simulink model "CryoDetHcd"  (R2016b)
settings: Solver=ode45  StartTime=0.0  StopTime=1e-3  RelTol=1e-3
PreLoadFcn:
  | setup_hcd
values from neighbouring files (symbols this model uses):
  A = sqrt(0.5*erfc(x))    [setup_hcd.m]
  etaRomData = zeros(1,128)    [setup_hcd.m]
  Fadc = 614e6    (= 614000000)    [setup_hcd.m]
  freqRomData = zeros(1,128)    [setup_hcd.m]
  freqRomData1 = zeros(1,128)    [setup_hcd.m]
  freqRomData2 = zeros(1,128)    [setup_hcd.m]
  freqRomData3 = zeros(1,128)    [setup_hcd.m]
undefined symbols (not defined in the file or in its folder): AXI4, B, C, D, j, Lite
libraries: xbsIndex_r4 x2151, CryoDetLibCMB x28, hdlsllib x8, dspsigops x2, simulink x1
(part 16 of 17)

== system CryoDetHcd/DspCore/DSP/channel_processor/channel_processor_x4/128_channel_processor3/Variant Subsystem/LMS/controller/1st_harmonic1/Subsystem1 ==
  note: D=2
  gain : Inport
  in : Inport  Port=2
  Mux : xbsIndex_r4/Mux  inputs=8  en=off  latency=1  precision=Full  arith_type=Unsigned  n_bits=16  bin_pt=14  quantization=Truncate  overflow=Wrap  dbl_ovrd=off  block_type=mux
  Shift2 : xbsIndex_r4/Shift  shift_dir=Right  shift_bits=13  en=off  latency=1  precision=User Defined  arith_type="Signed  (2's comp)"  n_bits=32  bin_pt=32  quantization=Truncate  overflow=Wrap  dbl_ovrd=off  block_type=shift
  Shift3 : xbsIndex_r4/Shift  shift_dir=Right  shift_bits=12  en=off  latency=1  precision=User Defined  arith_type="Signed  (2's comp)"  n_bits=32  bin_pt=32  quantization=Truncate  overflow=Wrap  dbl_ovrd=off  block_type=shift
  Shift4 : xbsIndex_r4/Shift  shift_dir=Right  shift_bits=6  en=off  latency=1  precision=User Defined  arith_type="Signed  (2's comp)"  n_bits=32  bin_pt=32  quantization=Truncate  overflow=Wrap  dbl_ovrd=off  block_type=shift
  Shift5 : xbsIndex_r4/Shift  shift_dir=Right  shift_bits=7  en=off  latency=1  precision=User Defined  arith_type="Signed  (2's comp)"  n_bits=32  bin_pt=32  quantization=Truncate  overflow=Wrap  dbl_ovrd=off  block_type=shift
  Shift6 : xbsIndex_r4/Shift  shift_dir=Right  shift_bits=8  en=off  latency=1  precision=User Defined  arith_type="Signed  (2's comp)"  n_bits=32  bin_pt=32  quantization=Truncate  overflow=Wrap  dbl_ovrd=off  block_type=shift
  Shift7 : xbsIndex_r4/Shift  shift_dir=Right  shift_bits=9  en=off  latency=1  precision=User Defined  arith_type="Signed  (2's comp)"  n_bits=32  bin_pt=32  quantization=Truncate  overflow=Wrap  dbl_ovrd=off  block_type=shift
  Shift8 : xbsIndex_r4/Shift  shift_dir=Right  shift_bits=10  en=off  latency=1  precision=User Defined  arith_type="Signed  (2's comp)"  n_bits=32  bin_pt=32  quantization=Truncate  overflow=Wrap  dbl_ovrd=off  block_type=shift
  Shift9 : xbsIndex_r4/Shift  shift_dir=Right  shift_bits=11  en=off  latency=1  precision=User Defined  arith_type="Signed  (2's comp)"  n_bits=32  bin_pt=32  quantization=Truncate  overflow=Wrap  dbl_ovrd=off  block_type=shift
  out : Outport
  wires:
  Shift4/1 -> Mux/9
  Shift5/1 -> Mux/8
  Shift6/1 -> Mux/7
  Shift7/1 -> Mux/6
  Shift8/1 -> Mux/5
  Shift9/1 -> Mux/4
  Shift3/1 -> Mux/3
  Shift2/1 -> Mux/2
  in/1 -> Shift2/1, Shift3/1, Shift9/1, Shift8/1, Shift7/1, Shift6/1, Shift5/1, Shift4/1
  Mux/1 -> out/1
  gain/1 -> Mux/1

== system CryoDetHcd/DspCore/DSP/channel_processor/channel_processor_x4/128_channel_processor3/Variant Subsystem/LMS/controller/1st_harmonic1/interleaved_accumulator1 ==
  note: D=5
  In1 : Inport
  enable : Inport  Port=2
  AddSub : xbsIndex_r4/AddSub  mode=Addition  use_carryin=off  use_carryout=off  en=off  latency=3  precision=User Defined  arith_type="Signed  (2's comp)"  n_bits=32  bin_pt=32  quantization=Truncate  overflow=Wrap  use_behavioral_HDL=off  hw_selection=Fabric  pipelined=off  dbl_ovrd=off  block_type=addsub
  Constant : xbsIndex_r4/Constant  const=0  gui_display_data_type=Fixed-point  arith_type=Signed (2's comp)  n_bits=32  bin_pt=32  preci_type=Single  exp_width=8  frac_width=24  explicit_period=off  period=1  equ=P=C  opselect=C  inp2=PCIN>>17  opr=+  inp1=P  carry=CIN  dbl_ovrd=off  block_type=constant
  Convert : xbsIndex_r4/Convert  gui_display_data_type=Fixed-point  arith_type="Signed  (2's comp)"  n_bits=28  bin_pt=28  float_type=Single  exp_bits=8  fraction_bits=24  quantization=Truncate  overflow=Wrap  en=off  latency=1  pipeline=off  dbl_ovrd=off  block_type=convert
  Delay : xbsIndex_r4/Delay  rst=off  infoeditControl=Selection of Reset will increase slice count due to use of real FFs and instead of SRLs  en=off  latency=124  reg_retiming=off  dbl_ovrd=off  block_type=delay
  Delay1 : xbsIndex_r4/Delay  rst=off  infoeditControl=Selection of Reset will increase slice count due to use of real FFs and instead of SRLs  en=off  latency=3  reg_retiming=off  dbl_ovrd=off  block_type=delay
  Mux : xbsIndex_r4/Mux  inputs=2  en=off  latency=1  precision=Full  arith_type=Unsigned  n_bits=16  bin_pt=14  quantization=Truncate  overflow=Wrap  dbl_ovrd=off  block_type=mux
  Out1 : Outport
  wires:
  In1/1 -> AddSub/1
  Delay/1 -> AddSub/2
  Convert/1 -> Out1/1
  Mux/1 -> Delay/1, Convert/1
  enable/1 -> Delay1/1
  Constant/1 -> Mux/2
  AddSub/1 -> Mux/3
  Delay1/1 -> Mux/1

== system CryoDetHcd/DspCore/DSP/channel_processor/channel_processor_x4/128_channel_processor3/Variant Subsystem/LMS/controller/1st_harmonic1/interleaved_accumulator2 ==
  In1 : Inport
  enable : Inport  Port=2
  AddSub : xbsIndex_r4/AddSub  mode=Addition  use_carryin=off  use_carryout=off  en=off  latency=3  precision=User Defined  arith_type="Signed  (2's comp)"  n_bits=32  bin_pt=32  quantization=Truncate  overflow=Wrap  use_behavioral_HDL=off  hw_selection=Fabric  pipelined=off  dbl_ovrd=off  block_type=addsub
  Constant : xbsIndex_r4/Constant  const=0  gui_display_data_type=Fixed-point  arith_type=Signed (2's comp)  n_bits=32  bin_pt=32  preci_type=Single  exp_width=8  frac_width=24  explicit_period=off  period=1  equ=P=C  opselect=C  inp2=PCIN>>17  opr=+  inp1=P  carry=CIN  dbl_ovrd=off  block_type=constant
  Convert : xbsIndex_r4/Convert  gui_display_data_type=Fixed-point  arith_type="Signed  (2's comp)"  n_bits=28  bin_pt=28  float_type=Single  exp_bits=8  fraction_bits=24  quantization=Truncate  overflow=Wrap  en=off  latency=1  pipeline=off  dbl_ovrd=off  block_type=convert
  Delay : xbsIndex_r4/Delay  rst=off  infoeditControl=Selection of Reset will increase slice count due to use of real FFs and instead of SRLs  en=off  latency=124  reg_retiming=off  dbl_ovrd=off  block_type=delay
  Delay1 : xbsIndex_r4/Delay  rst=off  infoeditControl=Selection of Reset will increase slice count due to use of real FFs and instead of SRLs  en=off  latency=3  reg_retiming=off  dbl_ovrd=off  block_type=delay
  Mux : xbsIndex_r4/Mux  inputs=2  en=off  latency=1  precision=Full  arith_type=Unsigned  n_bits=16  bin_pt=14  quantization=Truncate  overflow=Wrap  dbl_ovrd=off  block_type=mux
  Out1 : Outport
  wires:
  Delay1/1 -> Mux/1
  AddSub/1 -> Mux/3
  Constant/1 -> Mux/2
  enable/1 -> Delay1/1
  Mux/1 -> Convert/1, Delay/1
  Convert/1 -> Out1/1
  Delay/1 -> AddSub/2
  In1/1 -> AddSub/1

== system CryoDetHcd/DspCore/DSP/channel_processor/channel_processor_x4/128_channel_processor3/Variant Subsystem/LMS/controller/1st_harmonic2/Subsystem ==
  note: D=2
  gain : Inport
  in : Inport  Port=2
  Mux : xbsIndex_r4/Mux  inputs=8  en=off  latency=1  precision=Full  arith_type=Unsigned  n_bits=16  bin_pt=14  quantization=Truncate  overflow=Wrap  dbl_ovrd=off  block_type=mux
  Shift2 : xbsIndex_r4/Shift  shift_dir=Right  shift_bits=13  en=off  latency=1  precision=User Defined  arith_type="Signed  (2's comp)"  n_bits=32  bin_pt=32  quantization=Truncate  overflow=Wrap  dbl_ovrd=off  block_type=shift
  Shift3 : xbsIndex_r4/Shift  shift_dir=Right  shift_bits=12  en=off  latency=1  precision=User Defined  arith_type="Signed  (2's comp)"  n_bits=32  bin_pt=32  quantization=Truncate  overflow=Wrap  dbl_ovrd=off  block_type=shift
  Shift4 : xbsIndex_r4/Shift  shift_dir=Right  shift_bits=6  en=off  latency=1  precision=User Defined  arith_type="Signed  (2's comp)"  n_bits=32  bin_pt=32  quantization=Truncate  overflow=Wrap  dbl_ovrd=off  block_type=shift
  Shift5 : xbsIndex_r4/Shift  shift_dir=Right  shift_bits=7  en=off  latency=1  precision=User Defined  arith_type="Signed  (2's comp)"  n_bits=32  bin_pt=32  quantization=Truncate  overflow=Wrap  dbl_ovrd=off  block_type=shift
  Shift6 : xbsIndex_r4/Shift  shift_dir=Right  shift_bits=8  en=off  latency=1  precision=User Defined  arith_type="Signed  (2's comp)"  n_bits=32  bin_pt=32  quantization=Truncate  overflow=Wrap  dbl_ovrd=off  block_type=shift
  Shift7 : xbsIndex_r4/Shift  shift_dir=Right  shift_bits=9  en=off  latency=1  precision=User Defined  arith_type="Signed  (2's comp)"  n_bits=32  bin_pt=32  quantization=Truncate  overflow=Wrap  dbl_ovrd=off  block_type=shift
  Shift8 : xbsIndex_r4/Shift  shift_dir=Right  shift_bits=10  en=off  latency=1  precision=User Defined  arith_type="Signed  (2's comp)"  n_bits=32  bin_pt=32  quantization=Truncate  overflow=Wrap  dbl_ovrd=off  block_type=shift
  Shift9 : xbsIndex_r4/Shift  shift_dir=Right  shift_bits=11  en=off  latency=1  precision=User Defined  arith_type="Signed  (2's comp)"  n_bits=32  bin_pt=32  quantization=Truncate  overflow=Wrap  dbl_ovrd=off  block_type=shift
  out : Outport
  wires:
  Shift4/1 -> Mux/9
  Shift5/1 -> Mux/8
  Shift6/1 -> Mux/7
  Shift7/1 -> Mux/6
  Shift8/1 -> Mux/5
  Shift9/1 -> Mux/4
  Shift3/1 -> Mux/3
  Shift2/1 -> Mux/2
  in/1 -> Shift2/1, Shift3/1, Shift9/1, Shift8/1, Shift7/1, Shift6/1, Shift5/1, Shift4/1
  Mux/1 -> out/1
  gain/1 -> Mux/1

== system CryoDetHcd/DspCore/DSP/channel_processor/channel_processor_x4/128_channel_processor3/Variant Subsystem/LMS/controller/1st_harmonic2/Subsystem1 ==
  note: D=2
  gain : Inport
  in : Inport  Port=2
  Mux : xbsIndex_r4/Mux  inputs=8  en=off  latency=1  precision=Full  arith_type=Unsigned  n_bits=16  bin_pt=14  quantization=Truncate  overflow=Wrap  dbl_ovrd=off  block_type=mux
  Shift2 : xbsIndex_r4/Shift  shift_dir=Right  shift_bits=13  en=off  latency=1  precision=User Defined  arith_type="Signed  (2's comp)"  n_bits=32  bin_pt=32  quantization=Truncate  overflow=Wrap  dbl_ovrd=off  block_type=shift
  Shift3 : xbsIndex_r4/Shift  shift_dir=Right  shift_bits=12  en=off  latency=1  precision=User Defined  arith_type="Signed  (2's comp)"  n_bits=32  bin_pt=32  quantization=Truncate  overflow=Wrap  dbl_ovrd=off  block_type=shift
  Shift4 : xbsIndex_r4/Shift  shift_dir=Right  shift_bits=6  en=off  latency=1  precision=User Defined  arith_type="Signed  (2's comp)"  n_bits=32  bin_pt=32  quantization=Truncate  overflow=Wrap  dbl_ovrd=off  block_type=shift
  Shift5 : xbsIndex_r4/Shift  shift_dir=Right  shift_bits=7  en=off  latency=1  precision=User Defined  arith_type="Signed  (2's comp)"  n_bits=32  bin_pt=32  quantization=Truncate  overflow=Wrap  dbl_ovrd=off  block_type=shift
  Shift6 : xbsIndex_r4/Shift  shift_dir=Right  shift_bits=8  en=off  latency=1  precision=User Defined  arith_type="Signed  (2's comp)"  n_bits=32  bin_pt=32  quantization=Truncate  overflow=Wrap  dbl_ovrd=off  block_type=shift
  Shift7 : xbsIndex_r4/Shift  shift_dir=Right  shift_bits=9  en=off  latency=1  precision=User Defined  arith_type="Signed  (2's comp)"  n_bits=32  bin_pt=32  quantization=Truncate  overflow=Wrap  dbl_ovrd=off  block_type=shift
  Shift8 : xbsIndex_r4/Shift  shift_dir=Right  shift_bits=10  en=off  latency=1  precision=User Defined  arith_type="Signed  (2's comp)"  n_bits=32  bin_pt=32  quantization=Truncate  overflow=Wrap  dbl_ovrd=off  block_type=shift
  Shift9 : xbsIndex_r4/Shift  shift_dir=Right  shift_bits=11  en=off  latency=1  precision=User Defined  arith_type="Signed  (2's comp)"  n_bits=32  bin_pt=32  quantization=Truncate  overflow=Wrap  dbl_ovrd=off  block_type=shift
  out : Outport
  wires:
  gain/1 -> Mux/1
  Mux/1 -> out/1
  in/1 -> Shift4/1, Shift5/1, Shift6/1, Shift7/1, Shift8/1, Shift9/1, Shift3/1, Shift2/1
  Shift2/1 -> Mux/2
  Shift3/1 -> Mux/3
  Shift9/1 -> Mux/4
  Shift8/1 -> Mux/5
  Shift7/1 -> Mux/6
  Shift6/1 -> Mux/7
  Shift5/1 -> Mux/8
  Shift4/1 -> Mux/9

== system CryoDetHcd/DspCore/DSP/channel_processor/channel_processor_x4/128_channel_processor3/Variant Subsystem/LMS/controller/1st_harmonic2/interleaved_accumulator1 ==
  note: D=5
  In1 : Inport
  enable : Inport  Port=2
  AddSub : xbsIndex_r4/AddSub  mode=Addition  use_carryin=off  use_carryout=off  en=off  latency=3  precision=User Defined  arith_type="Signed  (2's comp)"  n_bits=32  bin_pt=32  quantization=Truncate  overflow=Wrap  use_behavioral_HDL=off  hw_selection=Fabric  pipelined=off  dbl_ovrd=off  block_type=addsub
  Constant : xbsIndex_r4/Constant  const=0  gui_display_data_type=Fixed-point  arith_type=Signed (2's comp)  n_bits=32  bin_pt=32  preci_type=Single  exp_width=8  frac_width=24  explicit_period=off  period=1  equ=P=C  opselect=C  inp2=PCIN>>17  opr=+  inp1=P  carry=CIN  dbl_ovrd=off  block_type=constant
  Convert : xbsIndex_r4/Convert  gui_display_data_type=Fixed-point  arith_type="Signed  (2's comp)"  n_bits=28  bin_pt=28  float_type=Single  exp_bits=8  fraction_bits=24  quantization=Truncate  overflow=Wrap  en=off  latency=1  pipeline=off  dbl_ovrd=off  block_type=convert
  Delay : xbsIndex_r4/Delay  rst=off  infoeditControl=Selection of Reset will increase slice count due to use of real FFs and instead of SRLs  en=off  latency=124  reg_retiming=off  dbl_ovrd=off  block_type=delay
  Delay1 : xbsIndex_r4/Delay  rst=off  infoeditControl=Selection of Reset will increase slice count due to use of real FFs and instead of SRLs  en=off  latency=3  reg_retiming=off  dbl_ovrd=off  block_type=delay
  Mux : xbsIndex_r4/Mux  inputs=2  en=off  latency=1  precision=Full  arith_type=Unsigned  n_bits=16  bin_pt=14  quantization=Truncate  overflow=Wrap  dbl_ovrd=off  block_type=mux
  Out1 : Outport
  wires:
  Delay1/1 -> Mux/1
  AddSub/1 -> Mux/3
  Constant/1 -> Mux/2
  enable/1 -> Delay1/1
  Mux/1 -> Convert/1, Delay/1
  Convert/1 -> Out1/1
  Delay/1 -> AddSub/2
  In1/1 -> AddSub/1

== system CryoDetHcd/DspCore/DSP/channel_processor/channel_processor_x4/128_channel_processor3/Variant Subsystem/LMS/controller/1st_harmonic2/interleaved_accumulator2 ==
  In1 : Inport
  enable : Inport  Port=2
  AddSub : xbsIndex_r4/AddSub  mode=Addition  use_carryin=off  use_carryout=off  en=off  latency=3  precision=User Defined  arith_type="Signed  (2's comp)"  n_bits=32  bin_pt=32  quantization=Truncate  overflow=Wrap  use_behavioral_HDL=off  hw_selection=Fabric  pipelined=off  dbl_ovrd=off  block_type=addsub
  Constant : xbsIndex_r4/Constant  const=0  gui_display_data_type=Fixed-point  arith_type=Signed (2's comp)  n_bits=32  bin_pt=32  preci_type=Single  exp_width=8  frac_width=24  explicit_period=off  period=1  equ=P=C  opselect=C  inp2=PCIN>>17  opr=+  inp1=P  carry=CIN  dbl_ovrd=off  block_type=constant
  Convert : xbsIndex_r4/Convert  gui_display_data_type=Fixed-point  arith_type="Signed  (2's comp)"  n_bits=28  bin_pt=28  float_type=Single  exp_bits=8  fraction_bits=24  quantization=Truncate  overflow=Wrap  en=off  latency=1  pipeline=off  dbl_ovrd=off  block_type=convert
  Delay : xbsIndex_r4/Delay  rst=off  infoeditControl=Selection of Reset will increase slice count due to use of real FFs and instead of SRLs  en=off  latency=124  reg_retiming=off  dbl_ovrd=off  block_type=delay
  Delay1 : xbsIndex_r4/Delay  rst=off  infoeditControl=Selection of Reset will increase slice count due to use of real FFs and instead of SRLs  en=off  latency=3  reg_retiming=off  dbl_ovrd=off  block_type=delay
  Mux : xbsIndex_r4/Mux  inputs=2  en=off  latency=1  precision=Full  arith_type=Unsigned  n_bits=16  bin_pt=14  quantization=Truncate  overflow=Wrap  dbl_ovrd=off  block_type=mux
  Out1 : Outport
  wires:
  In1/1 -> AddSub/1
  Delay/1 -> AddSub/2
  Convert/1 -> Out1/1
  Mux/1 -> Delay/1, Convert/1
  enable/1 -> Delay1/1
  Constant/1 -> Mux/2
  AddSub/1 -> Mux/3
  Delay1/1 -> Mux/1

== system CryoDetHcd/DspCore/DSP/channel_processor/channel_processor_x4/128_channel_processor3/Variant Subsystem/LMS/controller/DC/Subsystem ==
  note: D=2
  gain : Inport
  in : Inport  Port=2
  Mux : xbsIndex_r4/Mux  inputs=8  en=off  latency=1  precision=Full  arith_type=Unsigned  n_bits=16  bin_pt=14  quantization=Truncate  overflow=Wrap  dbl_ovrd=off  block_type=mux
  Shift2 : xbsIndex_r4/Shift  shift_dir=Right  shift_bits=13  en=off  latency=1  precision=User Defined  arith_type="Signed  (2's comp)"  n_bits=32  bin_pt=32  quantization=Truncate  overflow=Wrap  dbl_ovrd=off  block_type=shift
  Shift3 : xbsIndex_r4/Shift  shift_dir=Right  shift_bits=12  en=off  latency=1  precision=User Defined  arith_type="Signed  (2's comp)"  n_bits=32  bin_pt=32  quantization=Truncate  overflow=Wrap  dbl_ovrd=off  block_type=shift
  Shift4 : xbsIndex_r4/Shift  shift_dir=Right  shift_bits=6  en=off  latency=1  precision=User Defined  arith_type="Signed  (2's comp)"  n_bits=32  bin_pt=32  quantization=Truncate  overflow=Wrap  dbl_ovrd=off  block_type=shift
  Shift5 : xbsIndex_r4/Shift  shift_dir=Right  shift_bits=7  en=off  latency=1  precision=User Defined  arith_type="Signed  (2's comp)"  n_bits=32  bin_pt=32  quantization=Truncate  overflow=Wrap  dbl_ovrd=off  block_type=shift
  Shift6 : xbsIndex_r4/Shift  shift_dir=Right  shift_bits=8  en=off  latency=1  precision=User Defined  arith_type="Signed  (2's comp)"  n_bits=32  bin_pt=32  quantization=Truncate  overflow=Wrap  dbl_ovrd=off  block_type=shift
  Shift7 : xbsIndex_r4/Shift  shift_dir=Right  shift_bits=9  en=off  latency=1  precision=User Defined  arith_type="Signed  (2's comp)"  n_bits=32  bin_pt=32  quantization=Truncate  overflow=Wrap  dbl_ovrd=off  block_type=shift
  Shift8 : xbsIndex_r4/Shift  shift_dir=Right  shift_bits=10  en=off  latency=1  precision=User Defined  arith_type="Signed  (2's comp)"  n_bits=32  bin_pt=32  quantization=Truncate  overflow=Wrap  dbl_ovrd=off  block_type=shift
  Shift9 : xbsIndex_r4/Shift  shift_dir=Right  shift_bits=11  en=off  latency=1  precision=User Defined  arith_type="Signed  (2's comp)"  n_bits=32  bin_pt=32  quantization=Truncate  overflow=Wrap  dbl_ovrd=off  block_type=shift
  out : Outport
  wires:
  Shift4/1 -> Mux/9
  Shift5/1 -> Mux/8
  Shift6/1 -> Mux/7
  Shift7/1 -> Mux/6
  Shift8/1 -> Mux/5
  Shift9/1 -> Mux/4
  Shift3/1 -> Mux/3
  Shift2/1 -> Mux/2
  in/1 -> Shift2/1, Shift3/1, Shift9/1, Shift8/1, Shift7/1, Shift6/1, Shift5/1, Shift4/1
  Mux/1 -> out/1
  gain/1 -> Mux/1

== system CryoDetHcd/DspCore/DSP/channel_processor/channel_processor_x4/128_channel_processor3/Variant Subsystem/LMS/controller/DC/interleaved_accumulator2 ==
  In1 : Inport
  enable : Inport  Port=2
  AddSub : xbsIndex_r4/AddSub  mode=Addition  use_carryin=off  use_carryout=off  en=off  latency=3  precision=User Defined  arith_type="Signed  (2's comp)"  n_bits=32  bin_pt=32  quantization=Truncate  overflow=Wrap  use_behavioral_HDL=off  hw_selection=Fabric  pipelined=off  dbl_ovrd=off  block_type=addsub
  Constant : xbsIndex_r4/Constant  const=0  gui_display_data_type=Fixed-point  arith_type=Signed (2's comp)  n_bits=32  bin_pt=32  preci_type=Single  exp_width=8  frac_width=24  explicit_period=off  period=1  equ=P=C  opselect=C  inp2=PCIN>>17  opr=+  inp1=P  carry=CIN  dbl_ovrd=off  block_type=constant
  Convert : xbsIndex_r4/Convert  gui_display_data_type=Fixed-point  arith_type="Signed  (2's comp)"  n_bits=28  bin_pt=28  float_type=Single  exp_bits=8  fraction_bits=24  quantization=Truncate  overflow=Wrap  en=off  latency=1  pipeline=off  dbl_ovrd=off  block_type=convert
  Delay : xbsIndex_r4/Delay  rst=off  infoeditControl=Selection of Reset will increase slice count due to use of real FFs and instead of SRLs  en=off  latency=124  reg_retiming=off  dbl_ovrd=off  block_type=delay
  Delay1 : xbsIndex_r4/Delay  rst=off  infoeditControl=Selection of Reset will increase slice count due to use of real FFs and instead of SRLs  en=off  latency=3  reg_retiming=off  dbl_ovrd=off  block_type=delay
  Mux : xbsIndex_r4/Mux  inputs=2  en=off  latency=1  precision=Full  arith_type=Unsigned  n_bits=16  bin_pt=14  quantization=Truncate  overflow=Wrap  dbl_ovrd=off  block_type=mux
  Out1 : Outport
  wires:
  In1/1 -> AddSub/1
  Delay/1 -> AddSub/2
  Convert/1 -> Out1/1
  Mux/1 -> Delay/1, Convert/1
  enable/1 -> Delay1/1
  Constant/1 -> Mux/2
  AddSub/1 -> Mux/3
  Delay1/1 -> Mux/1

== system CryoDetHcd/DspCore/DSP/channel_processor/channel_processor_x4/128_channel_processor3/Variant Subsystem/LMS/controller/freqs/Subsystem ==
  Chan : Inport
  In2 : Inport  Port=2
  In3 : Inport  Port=3
  In4 : Inport  Port=4
  valid : Inport  Port=5
  Logical : xbsIndex_r4/Logical  logical_function=AND  inputs=2  en=off  latency=0  precision=Full  arith_type=Unsigned  n_bits=16  bin_pt=0  align_bp=on  dbl_ovrd=off  block_type=logical
  Register17 : xbsIndex_r4/Register  init=0  rst=off  en=on  dbl_ovrd=off  block_type=register
  Register18 : xbsIndex_r4/Register  init=0  rst=off  en=on  dbl_ovrd=off  block_type=register
  Relational : xbsIndex_r4/Relational  mode=a=b  op_type=Bool  en=off  latency=0  dbl_ovrd=off  block_type=relational
  Out2 : Outport
  Out3 : Outport  Port=2
  wires:
  Logical/1 -> Register17/2, Register18/2
  valid/1 -> Logical/2
  Relational/1 -> Logical/1
  In3/1 -> Register17/1
  In2/1 -> Relational/2
  Chan/1 -> Relational/1
  Register17/1 -> Out2/1
  Register18/1 -> Out3/1
  In4/1 -> Register18/1

== system CryoDetHcd/DspCore/DSP/channel_processor/channel_processor_x4/128_channel_processor3/Variant Subsystem/LMS/controller/freqs/Subsystem1 ==
  Chan : Inport
  In2 : Inport  Port=2
  In3 : Inport  Port=3
  In4 : Inport  Port=4
  valid : Inport  Port=5
  Logical : xbsIndex_r4/Logical  logical_function=AND  inputs=2  en=off  latency=0  precision=Full  arith_type=Unsigned  n_bits=16  bin_pt=0  align_bp=on  dbl_ovrd=off  block_type=logical
  Register17 : xbsIndex_r4/Register  init=0  rst=off  en=on  dbl_ovrd=off  block_type=register
  Register18 : xbsIndex_r4/Register  init=0  rst=off  en=on  dbl_ovrd=off  block_type=register
  Relational : xbsIndex_r4/Relational  mode=a=b  op_type=Bool  en=off  latency=0  dbl_ovrd=off  block_type=relational
  Out2 : Outport
  Out3 : Outport  Port=2
  wires:
  In4/1 -> Register18/1
  Register18/1 -> Out3/1
  Register17/1 -> Out2/1
  Chan/1 -> Relational/1
  In2/1 -> Relational/2
  In3/1 -> Register17/1
  Relational/1 -> Logical/1
  valid/1 -> Logical/2
  Logical/1 -> Register18/2, Register17/2

== system CryoDetHcd/DspCore/DSP/channel_processor/channel_processor_x4/128_channel_processor3/Variant Subsystem/LMS/controller/freqs/Subsystem2 ==
  Chan : Inport
  In2 : Inport  Port=2
  In3 : Inport  Port=3
  In4 : Inport  Port=4
  valid : Inport  Port=5
  Logical : xbsIndex_r4/Logical  logical_function=AND  inputs=2  en=off  latency=0  precision=Full  arith_type=Unsigned  n_bits=16  bin_pt=0  align_bp=on  dbl_ovrd=off  block_type=logical
  Register17 : xbsIndex_r4/Register  init=0  rst=off  en=on  dbl_ovrd=off  block_type=register
  Register18 : xbsIndex_r4/Register  init=0  rst=off  en=on  dbl_ovrd=off  block_type=register
  Relational : xbsIndex_r4/Relational  mode=a=b  op_type=Bool  en=off  latency=0  dbl_ovrd=off  block_type=relational
  Out2 : Outport
  Out3 : Outport  Port=2
  wires:
  Logical/1 -> Register17/2, Register18/2
  valid/1 -> Logical/2
  Relational/1 -> Logical/1
  In3/1 -> Register17/1
  In2/1 -> Relational/2
  Chan/1 -> Relational/1
  Register17/1 -> Out2/1
  Register18/1 -> Out3/1
  In4/1 -> Register18/1

== system CryoDetHcd/DspCore/DSP/channel_processor/channel_processor_x4/128_channel_processor4/Variant Subsystem/LMS/controller/1st_harmonic/Subsystem ==
  note: D=2
  gain : Inport
  in : Inport  Port=2
  Mux : xbsIndex_r4/Mux  inputs=8  en=off  latency=1  precision=Full  arith_type=Unsigned  n_bits=16  bin_pt=14  quantization=Truncate  overflow=Wrap  dbl_ovrd=off  block_type=mux
  Shift2 : xbsIndex_r4/Shift  shift_dir=Right  shift_bits=13  en=off  latency=1  precision=User Defined  arith_type="Signed  (2's comp)"  n_bits=32  bin_pt=32  quantization=Truncate  overflow=Wrap  dbl_ovrd=off  block_type=shift
  Shift3 : xbsIndex_r4/Shift  shift_dir=Right  shift_bits=12  en=off  latency=1  precision=User Defined  arith_type="Signed  (2's comp)"  n_bits=32  bin_pt=32  quantization=Truncate  overflow=Wrap  dbl_ovrd=off  block_type=shift
  Shift4 : xbsIndex_r4/Shift  shift_dir=Right  shift_bits=6  en=off  latency=1  precision=User Defined  arith_type="Signed  (2's comp)"  n_bits=32  bin_pt=32  quantization=Truncate  overflow=Wrap  dbl_ovrd=off  block_type=shift
  Shift5 : xbsIndex_r4/Shift  shift_dir=Right  shift_bits=7  en=off  latency=1  precision=User Defined  arith_type="Signed  (2's comp)"  n_bits=32  bin_pt=32  quantization=Truncate  overflow=Wrap  dbl_ovrd=off  block_type=shift
  Shift6 : xbsIndex_r4/Shift  shift_dir=Right  shift_bits=8  en=off  latency=1  precision=User Defined  arith_type="Signed  (2's comp)"  n_bits=32  bin_pt=32  quantization=Truncate  overflow=Wrap  dbl_ovrd=off  block_type=shift
  Shift7 : xbsIndex_r4/Shift  shift_dir=Right  shift_bits=9  en=off  latency=1  precision=User Defined  arith_type="Signed  (2's comp)"  n_bits=32  bin_pt=32  quantization=Truncate  overflow=Wrap  dbl_ovrd=off  block_type=shift
  Shift8 : xbsIndex_r4/Shift  shift_dir=Right  shift_bits=10  en=off  latency=1  precision=User Defined  arith_type="Signed  (2's comp)"  n_bits=32  bin_pt=32  quantization=Truncate  overflow=Wrap  dbl_ovrd=off  block_type=shift
  Shift9 : xbsIndex_r4/Shift  shift_dir=Right  shift_bits=11  en=off  latency=1  precision=User Defined  arith_type="Signed  (2's comp)"  n_bits=32  bin_pt=32  quantization=Truncate  overflow=Wrap  dbl_ovrd=off  block_type=shift
  out : Outport
  wires:
  gain/1 -> Mux/1
  Mux/1 -> out/1
  in/1 -> Shift4/1, Shift5/1, Shift6/1, Shift7/1, Shift8/1, Shift9/1, Shift3/1, Shift2/1
  Shift2/1 -> Mux/2
  Shift3/1 -> Mux/3
  Shift9/1 -> Mux/4
  Shift8/1 -> Mux/5
  Shift7/1 -> Mux/6
  Shift6/1 -> Mux/7
  Shift5/1 -> Mux/8
  Shift4/1 -> Mux/9

== system CryoDetHcd/DspCore/DSP/channel_processor/channel_processor_x4/128_channel_processor4/Variant Subsystem/LMS/controller/1st_harmonic/Subsystem1 ==
  note: D=2
  gain : Inport
  in : Inport  Port=2
  Mux : xbsIndex_r4/Mux  inputs=8  en=off  latency=1  precision=Full  arith_type=Unsigned  n_bits=16  bin_pt=14  quantization=Truncate  overflow=Wrap  dbl_ovrd=off  block_type=mux
  Shift2 : xbsIndex_r4/Shift  shift_dir=Right  shift_bits=13  en=off  latency=1  precision=User Defined  arith_type="Signed  (2's comp)"  n_bits=32  bin_pt=32  quantization=Truncate  overflow=Wrap  dbl_ovrd=off  block_type=shift
  Shift3 : xbsIndex_r4/Shift  shift_dir=Right  shift_bits=12  en=off  latency=1  precision=User Defined  arith_type="Signed  (2's comp)"  n_bits=32  bin_pt=32  quantization=Truncate  overflow=Wrap  dbl_ovrd=off  block_type=shift
  Shift4 : xbsIndex_r4/Shift  shift_dir=Right  shift_bits=6  en=off  latency=1  precision=User Defined  arith_type="Signed  (2's comp)"  n_bits=32  bin_pt=32  quantization=Truncate  overflow=Wrap  dbl_ovrd=off  block_type=shift
  Shift5 : xbsIndex_r4/Shift  shift_dir=Right  shift_bits=7  en=off  latency=1  precision=User Defined  arith_type="Signed  (2's comp)"  n_bits=32  bin_pt=32  quantization=Truncate  overflow=Wrap  dbl_ovrd=off  block_type=shift
  Shift6 : xbsIndex_r4/Shift  shift_dir=Right  shift_bits=8  en=off  latency=1  precision=User Defined  arith_type="Signed  (2's comp)"  n_bits=32  bin_pt=32  quantization=Truncate  overflow=Wrap  dbl_ovrd=off  block_type=shift
  Shift7 : xbsIndex_r4/Shift  shift_dir=Right  shift_bits=9  en=off  latency=1  precision=User Defined  arith_type="Signed  (2's comp)"  n_bits=32  bin_pt=32  quantization=Truncate  overflow=Wrap  dbl_ovrd=off  block_type=shift
  Shift8 : xbsIndex_r4/Shift  shift_dir=Right  shift_bits=10  en=off  latency=1  precision=User Defined  arith_type="Signed  (2's comp)"  n_bits=32  bin_pt=32  quantization=Truncate  overflow=Wrap  dbl_ovrd=off  block_type=shift
  Shift9 : xbsIndex_r4/Shift  shift_dir=Right  shift_bits=11  en=off  latency=1  precision=User Defined  arith_type="Signed  (2's comp)"  n_bits=32  bin_pt=32  quantization=Truncate  overflow=Wrap  dbl_ovrd=off  block_type=shift
  out : Outport
  wires:
  Shift4/1 -> Mux/9
  Shift5/1 -> Mux/8
  Shift6/1 -> Mux/7
  Shift7/1 -> Mux/6
  Shift8/1 -> Mux/5
  Shift9/1 -> Mux/4
  Shift3/1 -> Mux/3
  Shift2/1 -> Mux/2
  in/1 -> Shift2/1, Shift3/1, Shift9/1, Shift8/1, Shift7/1, Shift6/1, Shift5/1, Shift4/1
  Mux/1 -> out/1
  gain/1 -> Mux/1

== system CryoDetHcd/DspCore/DSP/channel_processor/channel_processor_x4/128_channel_processor4/Variant Subsystem/LMS/controller/1st_harmonic/interleaved_accumulator1 ==
  note: D=5
  In1 : Inport
  enable : Inport  Port=2
  AddSub : xbsIndex_r4/AddSub  mode=Addition  use_carryin=off  use_carryout=off  en=off  latency=3  precision=User Defined  arith_type="Signed  (2's comp)"  n_bits=32  bin_pt=32  quantization=Truncate  overflow=Wrap  use_behavioral_HDL=off  hw_selection=Fabric  pipelined=off  dbl_ovrd=off  block_type=addsub
  Constant : xbsIndex_r4/Constant  const=0  gui_display_data_type=Fixed-point  arith_type=Signed (2's comp)  n_bits=32  bin_pt=32  preci_type=Single  exp_width=8  frac_width=24  explicit_period=off  period=1  equ=P=C  opselect=C  inp2=PCIN>>17  opr=+  inp1=P  carry=CIN  dbl_ovrd=off  block_type=constant
  Convert : xbsIndex_r4/Convert  gui_display_data_type=Fixed-point  arith_type="Signed  (2's comp)"  n_bits=28  bin_pt=28  float_type=Single  exp_bits=8  fraction_bits=24  quantization=Truncate  overflow=Wrap  en=off  latency=1  pipeline=off  dbl_ovrd=off  block_type=convert
  Delay : xbsIndex_r4/Delay  rst=off  infoeditControl=Selection of Reset will increase slice count due to use of real FFs and instead of SRLs  en=off  latency=124  reg_retiming=off  dbl_ovrd=off  block_type=delay
  Delay1 : xbsIndex_r4/Delay  rst=off  infoeditControl=Selection of Reset will increase slice count due to use of real FFs and instead of SRLs  en=off  latency=3  reg_retiming=off  dbl_ovrd=off  block_type=delay
  Mux : xbsIndex_r4/Mux  inputs=2  en=off  latency=1  precision=Full  arith_type=Unsigned  n_bits=16  bin_pt=14  quantization=Truncate  overflow=Wrap  dbl_ovrd=off  block_type=mux
  Out1 : Outport
  wires:
  In1/1 -> AddSub/1
  Delay/1 -> AddSub/2
  Convert/1 -> Out1/1
  Mux/1 -> Delay/1, Convert/1
  enable/1 -> Delay1/1
  Constant/1 -> Mux/2
  AddSub/1 -> Mux/3
  Delay1/1 -> Mux/1

== system CryoDetHcd/DspCore/DSP/channel_processor/channel_processor_x4/128_channel_processor4/Variant Subsystem/LMS/controller/1st_harmonic/interleaved_accumulator2 ==
  In1 : Inport
  enable : Inport  Port=2
  AddSub : xbsIndex_r4/AddSub  mode=Addition  use_carryin=off  use_carryout=off  en=off  latency=3  precision=User Defined  arith_type="Signed  (2's comp)"  n_bits=32  bin_pt=32  quantization=Truncate  overflow=Wrap  use_behavioral_HDL=off  hw_selection=Fabric  pipelined=off  dbl_ovrd=off  block_type=addsub
  Constant : xbsIndex_r4/Constant  const=0  gui_display_data_type=Fixed-point  arith_type=Signed (2's comp)  n_bits=32  bin_pt=32  preci_type=Single  exp_width=8  frac_width=24  explicit_period=off  period=1  equ=P=C  opselect=C  inp2=PCIN>>17  opr=+  inp1=P  carry=CIN  dbl_ovrd=off  block_type=constant
  Convert : xbsIndex_r4/Convert  gui_display_data_type=Fixed-point  arith_type="Signed  (2's comp)"  n_bits=28  bin_pt=28  float_type=Single  exp_bits=8  fraction_bits=24  quantization=Truncate  overflow=Wrap  en=off  latency=1  pipeline=off  dbl_ovrd=off  block_type=convert
  Delay : xbsIndex_r4/Delay  rst=off  infoeditControl=Selection of Reset will increase slice count due to use of real FFs and instead of SRLs  en=off  latency=124  reg_retiming=off  dbl_ovrd=off  block_type=delay
  Delay1 : xbsIndex_r4/Delay  rst=off  infoeditControl=Selection of Reset will increase slice count due to use of real FFs and instead of SRLs  en=off  latency=3  reg_retiming=off  dbl_ovrd=off  block_type=delay
  Mux : xbsIndex_r4/Mux  inputs=2  en=off  latency=1  precision=Full  arith_type=Unsigned  n_bits=16  bin_pt=14  quantization=Truncate  overflow=Wrap  dbl_ovrd=off  block_type=mux
  Out1 : Outport
  wires:
  Delay1/1 -> Mux/1
  AddSub/1 -> Mux/3
  Constant/1 -> Mux/2
  enable/1 -> Delay1/1
  Mux/1 -> Convert/1, Delay/1
  Convert/1 -> Out1/1
  Delay/1 -> AddSub/2
  In1/1 -> AddSub/1

== system CryoDetHcd/DspCore/DSP/channel_processor/channel_processor_x4/128_channel_processor4/Variant Subsystem/LMS/controller/1st_harmonic1/Subsystem ==
  note: D=2
  gain : Inport
  in : Inport  Port=2
  Mux : xbsIndex_r4/Mux  inputs=8  en=off  latency=1  precision=Full  arith_type=Unsigned  n_bits=16  bin_pt=14  quantization=Truncate  overflow=Wrap  dbl_ovrd=off  block_type=mux
  Shift2 : xbsIndex_r4/Shift  shift_dir=Right  shift_bits=13  en=off  latency=1  precision=User Defined  arith_type="Signed  (2's comp)"  n_bits=32  bin_pt=32  quantization=Truncate  overflow=Wrap  dbl_ovrd=off  block_type=shift
  Shift3 : xbsIndex_r4/Shift  shift_dir=Right  shift_bits=12  en=off  latency=1  precision=User Defined  arith_type="Signed  (2's comp)"  n_bits=32  bin_pt=32  quantization=Truncate  overflow=Wrap  dbl_ovrd=off  block_type=shift
  Shift4 : xbsIndex_r4/Shift  shift_dir=Right  shift_bits=6  en=off  latency=1  precision=User Defined  arith_type="Signed  (2's comp)"  n_bits=32  bin_pt=32  quantization=Truncate  overflow=Wrap  dbl_ovrd=off  block_type=shift
  Shift5 : xbsIndex_r4/Shift  shift_dir=Right  shift_bits=7  en=off  latency=1  precision=User Defined  arith_type="Signed  (2's comp)"  n_bits=32  bin_pt=32  quantization=Truncate  overflow=Wrap  dbl_ovrd=off  block_type=shift
  Shift6 : xbsIndex_r4/Shift  shift_dir=Right  shift_bits=8  en=off  latency=1  precision=User Defined  arith_type="Signed  (2's comp)"  n_bits=32  bin_pt=32  quantization=Truncate  overflow=Wrap  dbl_ovrd=off  block_type=shift
  Shift7 : xbsIndex_r4/Shift  shift_dir=Right  shift_bits=9  en=off  latency=1  precision=User Defined  arith_type="Signed  (2's comp)"  n_bits=32  bin_pt=32  quantization=Truncate  overflow=Wrap  dbl_ovrd=off  block_type=shift
  Shift8 : xbsIndex_r4/Shift  shift_dir=Right  shift_bits=10  en=off  latency=1  precision=User Defined  arith_type="Signed  (2's comp)"  n_bits=32  bin_pt=32  quantization=Truncate  overflow=Wrap  dbl_ovrd=off  block_type=shift
  Shift9 : xbsIndex_r4/Shift  shift_dir=Right  shift_bits=11  en=off  latency=1  precision=User Defined  arith_type="Signed  (2's comp)"  n_bits=32  bin_pt=32  quantization=Truncate  overflow=Wrap  dbl_ovrd=off  block_type=shift
  out : Outport
  wires:
  Shift4/1 -> Mux/9
  Shift5/1 -> Mux/8
  Shift6/1 -> Mux/7
  Shift7/1 -> Mux/6
  Shift8/1 -> Mux/5
  Shift9/1 -> Mux/4
  Shift3/1 -> Mux/3
  Shift2/1 -> Mux/2
  in/1 -> Shift2/1, Shift3/1, Shift9/1, Shift8/1, Shift7/1, Shift6/1, Shift5/1, Shift4/1
  Mux/1 -> out/1
  gain/1 -> Mux/1

== system CryoDetHcd/DspCore/DSP/channel_processor/channel_processor_x4/128_channel_processor4/Variant Subsystem/LMS/controller/1st_harmonic1/Subsystem1 ==
  note: D=2
  gain : Inport
  in : Inport  Port=2
  Mux : xbsIndex_r4/Mux  inputs=8  en=off  latency=1  precision=Full  arith_type=Unsigned  n_bits=16  bin_pt=14  quantization=Truncate  overflow=Wrap  dbl_ovrd=off  block_type=mux
  Shift2 : xbsIndex_r4/Shift  shift_dir=Right  shift_bits=13  en=off  latency=1  precision=User Defined  arith_type="Signed  (2's comp)"  n_bits=32  bin_pt=32  quantization=Truncate  overflow=Wrap  dbl_ovrd=off  block_type=shift
  Shift3 : xbsIndex_r4/Shift  shift_dir=Right  shift_bits=12  en=off  latency=1  precision=User Defined  arith_type="Signed  (2's comp)"  n_bits=32  bin_pt=32  quantization=Truncate  overflow=Wrap  dbl_ovrd=off  block_type=shift
  Shift4 : xbsIndex_r4/Shift  shift_dir=Right  shift_bits=6  en=off  latency=1  precision=User Defined  arith_type="Signed  (2's comp)"  n_bits=32  bin_pt=32  quantization=Truncate  overflow=Wrap  dbl_ovrd=off  block_type=shift
  Shift5 : xbsIndex_r4/Shift  shift_dir=Right  shift_bits=7  en=off  latency=1  precision=User Defined  arith_type="Signed  (2's comp)"  n_bits=32  bin_pt=32  quantization=Truncate  overflow=Wrap  dbl_ovrd=off  block_type=shift
  Shift6 : xbsIndex_r4/Shift  shift_dir=Right  shift_bits=8  en=off  latency=1  precision=User Defined  arith_type="Signed  (2's comp)"  n_bits=32  bin_pt=32  quantization=Truncate  overflow=Wrap  dbl_ovrd=off  block_type=shift
  Shift7 : xbsIndex_r4/Shift  shift_dir=Right  shift_bits=9  en=off  latency=1  precision=User Defined  arith_type="Signed  (2's comp)"  n_bits=32  bin_pt=32  quantization=Truncate  overflow=Wrap  dbl_ovrd=off  block_type=shift
  Shift8 : xbsIndex_r4/Shift  shift_dir=Right  shift_bits=10  en=off  latency=1  precision=User Defined  arith_type="Signed  (2's comp)"  n_bits=32  bin_pt=32  quantization=Truncate  overflow=Wrap  dbl_ovrd=off  block_type=shift
  Shift9 : xbsIndex_r4/Shift  shift_dir=Right  shift_bits=11  en=off  latency=1  precision=User Defined  arith_type="Signed  (2's comp)"  n_bits=32  bin_pt=32  quantization=Truncate  overflow=Wrap  dbl_ovrd=off  block_type=shift
  out : Outport
  wires:
  gain/1 -> Mux/1
  Mux/1 -> out/1
  in/1 -> Shift4/1, Shift5/1, Shift6/1, Shift7/1, Shift8/1, Shift9/1, Shift3/1, Shift2/1
  Shift2/1 -> Mux/2
  Shift3/1 -> Mux/3
  Shift9/1 -> Mux/4
  Shift8/1 -> Mux/5
  Shift7/1 -> Mux/6
  Shift6/1 -> Mux/7
  Shift5/1 -> Mux/8
  Shift4/1 -> Mux/9

== system CryoDetHcd/DspCore/DSP/channel_processor/channel_processor_x4/128_channel_processor4/Variant Subsystem/LMS/controller/1st_harmonic1/interleaved_accumulator1 ==
  note: D=5
  In1 : Inport
  enable : Inport  Port=2
  AddSub : xbsIndex_r4/AddSub  mode=Addition  use_carryin=off  use_carryout=off  en=off  latency=3  precision=User Defined  arith_type="Signed  (2's comp)"  n_bits=32  bin_pt=32  quantization=Truncate  overflow=Wrap  use_behavioral_HDL=off  hw_selection=Fabric  pipelined=off  dbl_ovrd=off  block_type=addsub
  Constant : xbsIndex_r4/Constant  const=0  gui_display_data_type=Fixed-point  arith_type=Signed (2's comp)  n_bits=32  bin_pt=32  preci_type=Single  exp_width=8  frac_width=24  explicit_period=off  period=1  equ=P=C  opselect=C  inp2=PCIN>>17  opr=+  inp1=P  carry=CIN  dbl_ovrd=off  block_type=constant
  Convert : xbsIndex_r4/Convert  gui_display_data_type=Fixed-point  arith_type="Signed  (2's comp)"  n_bits=28  bin_pt=28  float_type=Single  exp_bits=8  fraction_bits=24  quantization=Truncate  overflow=Wrap  en=off  latency=1  pipeline=off  dbl_ovrd=off  block_type=convert
  Delay : xbsIndex_r4/Delay  rst=off  infoeditControl=Selection of Reset will increase slice count due to use of real FFs and instead of SRLs  en=off  latency=124  reg_retiming=off  dbl_ovrd=off  block_type=delay
  Delay1 : xbsIndex_r4/Delay  rst=off  infoeditControl=Selection of Reset will increase slice count due to use of real FFs and instead of SRLs  en=off  latency=3  reg_retiming=off  dbl_ovrd=off  block_type=delay
  Mux : xbsIndex_r4/Mux  inputs=2  en=off  latency=1  precision=Full  arith_type=Unsigned  n_bits=16  bin_pt=14  quantization=Truncate  overflow=Wrap  dbl_ovrd=off  block_type=mux
  Out1 : Outport
  wires:
  Delay1/1 -> Mux/1
  AddSub/1 -> Mux/3
  Constant/1 -> Mux/2
  enable/1 -> Delay1/1
  Mux/1 -> Convert/1, Delay/1
  Convert/1 -> Out1/1
  Delay/1 -> AddSub/2
  In1/1 -> AddSub/1

== system CryoDetHcd/DspCore/DSP/channel_processor/channel_processor_x4/128_channel_processor4/Variant Subsystem/LMS/controller/1st_harmonic1/interleaved_accumulator2 ==
  In1 : Inport
  enable : Inport  Port=2
  AddSub : xbsIndex_r4/AddSub  mode=Addition  use_carryin=off  use_carryout=off  en=off  latency=3  precision=User Defined  arith_type="Signed  (2's comp)"  n_bits=32  bin_pt=32  quantization=Truncate  overflow=Wrap  use_behavioral_HDL=off  hw_selection=Fabric  pipelined=off  dbl_ovrd=off  block_type=addsub
  Constant : xbsIndex_r4/Constant  const=0  gui_display_data_type=Fixed-point  arith_type=Signed (2's comp)  n_bits=32  bin_pt=32  preci_type=Single  exp_width=8  frac_width=24  explicit_period=off  period=1  equ=P=C  opselect=C  inp2=PCIN>>17  opr=+  inp1=P  carry=CIN  dbl_ovrd=off  block_type=constant
  Convert : xbsIndex_r4/Convert  gui_display_data_type=Fixed-point  arith_type="Signed  (2's comp)"  n_bits=28  bin_pt=28  float_type=Single  exp_bits=8  fraction_bits=24  quantization=Truncate  overflow=Wrap  en=off  latency=1  pipeline=off  dbl_ovrd=off  block_type=convert
  Delay : xbsIndex_r4/Delay  rst=off  infoeditControl=Selection of Reset will increase slice count due to use of real FFs and instead of SRLs  en=off  latency=124  reg_retiming=off  dbl_ovrd=off  block_type=delay
  Delay1 : xbsIndex_r4/Delay  rst=off  infoeditControl=Selection of Reset will increase slice count due to use of real FFs and instead of SRLs  en=off  latency=3  reg_retiming=off  dbl_ovrd=off  block_type=delay
  Mux : xbsIndex_r4/Mux  inputs=2  en=off  latency=1  precision=Full  arith_type=Unsigned  n_bits=16  bin_pt=14  quantization=Truncate  overflow=Wrap  dbl_ovrd=off  block_type=mux
  Out1 : Outport
  wires:
  In1/1 -> AddSub/1
  Delay/1 -> AddSub/2
  Convert/1 -> Out1/1
  Mux/1 -> Delay/1, Convert/1
  enable/1 -> Delay1/1
  Constant/1 -> Mux/2
  AddSub/1 -> Mux/3
  Delay1/1 -> Mux/1

== system CryoDetHcd/DspCore/DSP/channel_processor/channel_processor_x4/128_channel_processor4/Variant Subsystem/LMS/controller/1st_harmonic2/Subsystem ==
  note: D=2
  gain : Inport
  in : Inport  Port=2
  Mux : xbsIndex_r4/Mux  inputs=8  en=off  latency=1  precision=Full  arith_type=Unsigned  n_bits=16  bin_pt=14  quantization=Truncate  overflow=Wrap  dbl_ovrd=off  block_type=mux
  Shift2 : xbsIndex_r4/Shift  shift_dir=Right  shift_bits=13  en=off  latency=1  precision=User Defined  arith_type="Signed  (2's comp)"  n_bits=32  bin_pt=32  quantization=Truncate  overflow=Wrap  dbl_ovrd=off  block_type=shift
  Shift3 : xbsIndex_r4/Shift  shift_dir=Right  shift_bits=12  en=off  latency=1  precision=User Defined  arith_type="Signed  (2's comp)"  n_bits=32  bin_pt=32  quantization=Truncate  overflow=Wrap  dbl_ovrd=off  block_type=shift
  Shift4 : xbsIndex_r4/Shift  shift_dir=Right  shift_bits=6  en=off  latency=1  precision=User Defined  arith_type="Signed  (2's comp)"  n_bits=32  bin_pt=32  quantization=Truncate  overflow=Wrap  dbl_ovrd=off  block_type=shift
  Shift5 : xbsIndex_r4/Shift  shift_dir=Right  shift_bits=7  en=off  latency=1  precision=User Defined  arith_type="Signed  (2's comp)"  n_bits=32  bin_pt=32  quantization=Truncate  overflow=Wrap  dbl_ovrd=off  block_type=shift
  Shift6 : xbsIndex_r4/Shift  shift_dir=Right  shift_bits=8  en=off  latency=1  precision=User Defined  arith_type="Signed  (2's comp)"  n_bits=32  bin_pt=32  quantization=Truncate  overflow=Wrap  dbl_ovrd=off  block_type=shift
  Shift7 : xbsIndex_r4/Shift  shift_dir=Right  shift_bits=9  en=off  latency=1  precision=User Defined  arith_type="Signed  (2's comp)"  n_bits=32  bin_pt=32  quantization=Truncate  overflow=Wrap  dbl_ovrd=off  block_type=shift
  Shift8 : xbsIndex_r4/Shift  shift_dir=Right  shift_bits=10  en=off  latency=1  precision=User Defined  arith_type="Signed  (2's comp)"  n_bits=32  bin_pt=32  quantization=Truncate  overflow=Wrap  dbl_ovrd=off  block_type=shift
  Shift9 : xbsIndex_r4/Shift  shift_dir=Right  shift_bits=11  en=off  latency=1  precision=User Defined  arith_type="Signed  (2's comp)"  n_bits=32  bin_pt=32  quantization=Truncate  overflow=Wrap  dbl_ovrd=off  block_type=shift
  out : Outport
  wires:
  gain/1 -> Mux/1
  Mux/1 -> out/1
  in/1 -> Shift4/1, Shift5/1, Shift6/1, Shift7/1, Shift8/1, Shift9/1, Shift3/1, Shift2/1
  Shift2/1 -> Mux/2
  Shift3/1 -> Mux/3
  Shift9/1 -> Mux/4
  Shift8/1 -> Mux/5
  Shift7/1 -> Mux/6
  Shift6/1 -> Mux/7
  Shift5/1 -> Mux/8
  Shift4/1 -> Mux/9

== system CryoDetHcd/DspCore/DSP/channel_processor/channel_processor_x4/128_channel_processor4/Variant Subsystem/LMS/controller/1st_harmonic2/Subsystem1 ==
  note: D=2
  gain : Inport
  in : Inport  Port=2
  Mux : xbsIndex_r4/Mux  inputs=8  en=off  latency=1  precision=Full  arith_type=Unsigned  n_bits=16  bin_pt=14  quantization=Truncate  overflow=Wrap  dbl_ovrd=off  block_type=mux
  Shift2 : xbsIndex_r4/Shift  shift_dir=Right  shift_bits=13  en=off  latency=1  precision=User Defined  arith_type="Signed  (2's comp)"  n_bits=32  bin_pt=32  quantization=Truncate  overflow=Wrap  dbl_ovrd=off  block_type=shift
  Shift3 : xbsIndex_r4/Shift  shift_dir=Right  shift_bits=12  en=off  latency=1  precision=User Defined  arith_type="Signed  (2's comp)"  n_bits=32  bin_pt=32  quantization=Truncate  overflow=Wrap  dbl_ovrd=off  block_type=shift
  Shift4 : xbsIndex_r4/Shift  shift_dir=Right  shift_bits=6  en=off  latency=1  precision=User Defined  arith_type="Signed  (2's comp)"  n_bits=32  bin_pt=32  quantization=Truncate  overflow=Wrap  dbl_ovrd=off  block_type=shift
  Shift5 : xbsIndex_r4/Shift  shift_dir=Right  shift_bits=7  en=off  latency=1  precision=User Defined  arith_type="Signed  (2's comp)"  n_bits=32  bin_pt=32  quantization=Truncate  overflow=Wrap  dbl_ovrd=off  block_type=shift
  Shift6 : xbsIndex_r4/Shift  shift_dir=Right  shift_bits=8  en=off  latency=1  precision=User Defined  arith_type="Signed  (2's comp)"  n_bits=32  bin_pt=32  quantization=Truncate  overflow=Wrap  dbl_ovrd=off  block_type=shift
  Shift7 : xbsIndex_r4/Shift  shift_dir=Right  shift_bits=9  en=off  latency=1  precision=User Defined  arith_type="Signed  (2's comp)"  n_bits=32  bin_pt=32  quantization=Truncate  overflow=Wrap  dbl_ovrd=off  block_type=shift
  Shift8 : xbsIndex_r4/Shift  shift_dir=Right  shift_bits=10  en=off  latency=1  precision=User Defined  arith_type="Signed  (2's comp)"  n_bits=32  bin_pt=32  quantization=Truncate  overflow=Wrap  dbl_ovrd=off  block_type=shift
  Shift9 : xbsIndex_r4/Shift  shift_dir=Right  shift_bits=11  en=off  latency=1  precision=User Defined  arith_type="Signed  (2's comp)"  n_bits=32  bin_pt=32  quantization=Truncate  overflow=Wrap  dbl_ovrd=off  block_type=shift
  out : Outport
  wires:
  Shift4/1 -> Mux/9
  Shift5/1 -> Mux/8
  Shift6/1 -> Mux/7
  Shift7/1 -> Mux/6
  Shift8/1 -> Mux/5
  Shift9/1 -> Mux/4
  Shift3/1 -> Mux/3
  Shift2/1 -> Mux/2
  in/1 -> Shift2/1, Shift3/1, Shift9/1, Shift8/1, Shift7/1, Shift6/1, Shift5/1, Shift4/1
  Mux/1 -> out/1
  gain/1 -> Mux/1

== system CryoDetHcd/DspCore/DSP/channel_processor/channel_processor_x4/128_channel_processor4/Variant Subsystem/LMS/controller/1st_harmonic2/interleaved_accumulator1 ==
  note: D=5
  In1 : Inport
  enable : Inport  Port=2
  AddSub : xbsIndex_r4/AddSub  mode=Addition  use_carryin=off  use_carryout=off  en=off  latency=3  precision=User Defined  arith_type="Signed  (2's comp)"  n_bits=32  bin_pt=32  quantization=Truncate  overflow=Wrap  use_behavioral_HDL=off  hw_selection=Fabric  pipelined=off  dbl_ovrd=off  block_type=addsub
  Constant : xbsIndex_r4/Constant  const=0  gui_display_data_type=Fixed-point  arith_type=Signed (2's comp)  n_bits=32  bin_pt=32  preci_type=Single  exp_width=8  frac_width=24  explicit_period=off  period=1  equ=P=C  opselect=C  inp2=PCIN>>17  opr=+  inp1=P  carry=CIN  dbl_ovrd=off  block_type=constant
  Convert : xbsIndex_r4/Convert  gui_display_data_type=Fixed-point  arith_type="Signed  (2's comp)"  n_bits=28  bin_pt=28  float_type=Single  exp_bits=8  fraction_bits=24  quantization=Truncate  overflow=Wrap  en=off  latency=1  pipeline=off  dbl_ovrd=off  block_type=convert
  Delay : xbsIndex_r4/Delay  rst=off  infoeditControl=Selection of Reset will increase slice count due to use of real FFs and instead of SRLs  en=off  latency=124  reg_retiming=off  dbl_ovrd=off  block_type=delay
  Delay1 : xbsIndex_r4/Delay  rst=off  infoeditControl=Selection of Reset will increase slice count due to use of real FFs and instead of SRLs  en=off  latency=3  reg_retiming=off  dbl_ovrd=off  block_type=delay
  Mux : xbsIndex_r4/Mux  inputs=2  en=off  latency=1  precision=Full  arith_type=Unsigned  n_bits=16  bin_pt=14  quantization=Truncate  overflow=Wrap  dbl_ovrd=off  block_type=mux
  Out1 : Outport
  wires:
  In1/1 -> AddSub/1
  Delay/1 -> AddSub/2
  Convert/1 -> Out1/1
  Mux/1 -> Delay/1, Convert/1
  enable/1 -> Delay1/1
  Constant/1 -> Mux/2
  AddSub/1 -> Mux/3
  Delay1/1 -> Mux/1
